simulink model "pid_ctrl_sim"  (R2015a)
settings: Solver=ode45  StartTime=0.0  StopTime=6  RelTol=1e-3
libraries: simulink x1
settings Model: Creator=rojas-j  LastModifiedBy=root

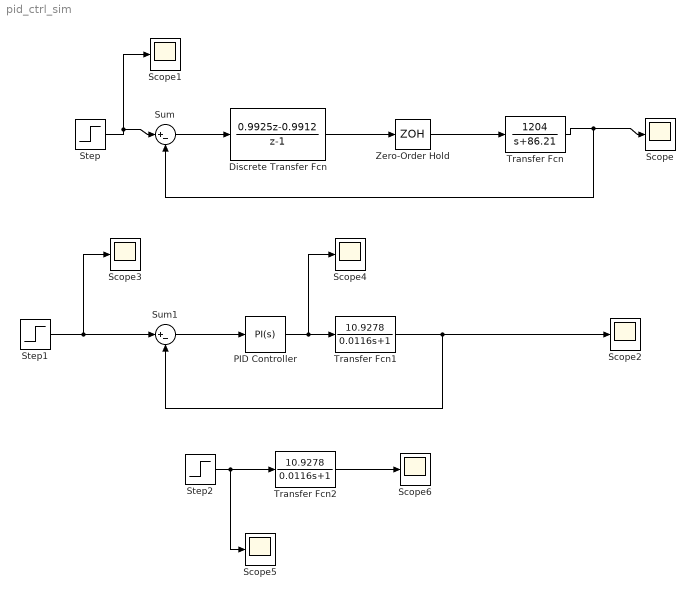
== system pid_ctrl_sim ==
  Discrete Transfer Fcn : DiscreteTransferFcn  Numerator=[0.9925,-0.9912]  Denominator=[1, -1]  SampleTime=0.00116
  PID Controller : simulink/Continuous/PID Controller  Controller=PI  TimeDomain=Continuous-time  SampleTime=-1  IntegratorMethod=Forward Euler  FilterMethod=Forward Euler  Form=Parallel  UseFilter=on  ControllerParametersSource=internal  P=0.99  I=1.17  D=0  N=100  InitialConditionSource=internal  InitialConditionForIntegrator=0  InitialConditionForFilter=0  ExternalReset=none  LimitOutput=off  UpperSaturationLimit=100  LowerSaturationLimit=0  LinearizeAsGain=on  AntiWindupMode=none  Kb=1  TrackingMode=off  Kt=1  PParamMin=[]  PParamMax=[]  IParamMin=[]  IParamMax=[]  DParamMin=[]  DParamMax=[]  NParamMin=[]  NParamMax=[]  KbParamMin=[]  KbParamMax=[]  KtParamMin=[]  KtParamMax=[]  POutMin=[]  POutMax=[]  IOutMin=[]  IOutMax=[]  DOutMin=[]  DOutMax=[]  NOutMin=[]  NOutMax=[]  KbOutMin=[]  KbOutMax=[]  KtOutMin=[]  KtOutMax=[]  IntegratorOutMin=[]  IntegratorOutMax=[]  FilterOutMin=[]  FilterOutMax=[]  SumOutMin=[]  SumOutMax=[]  SumI1OutMin=[]  SumI1OutMax=[]  SumI2OutMin=[]  SumI2OutMax=[]  SumI3OutMin=[]  SumI3OutMax=[]  SumDOutMin=[]  SumDOutMax=[]  SaturationOutMin=[]  SaturationOutMax=[]  IntegratorContinuousStateAttributes=''  IntegratorStateMustResolveToSignalObject=off  IntegratorRTWStateStorageClass=Auto  FilterContinuousStateAttributes=''  FilterStateMustResolveToSignalObject=off  FilterRTWStateStorageClass=Auto  DifferentiatorICPrevScaledInput=0  DifferentiatorOutMin=[]  DifferentiatorOutMax=[]
  Scope{,1..6} (7 alike) : Scope
      Scope2 settings: YMin=-1  YMax=1  SaveName=ScopeData2
      Scope3 settings: SaveName=ScopeData3
      Scope4 settings: YMin=-1  YMax=1  SaveName=ScopeData4
      Scope5 settings: SaveName=ScopeData5
      Scope6 settings: YMin=-1  YMax=1  SaveName=ScopeData6
  Step : Step  SampleTime=0.1
  Step1 : Step  After=500  SampleTime=0.1
  Step2 : Step  After=50  SampleTime=0.1
  Sum : Sum  Inputs=|+-
  Sum1 : Sum  Inputs=|+-
  Transfer Fcn : TransferFcn  Numerator=[1204]  Denominator=[1 86.21]
  Transfer Fcn1 : TransferFcn  Numerator=[10.9278]  Denominator=[0.0116 1]
  Transfer Fcn2 : TransferFcn  Numerator=[10.9278]  Denominator=[0.0116 1]
  Zero-Order Hold : ZeroOrderHold  SampleTime=0.00116
  wires:
  Step/1 -> Scope1/1, Sum/1
  Sum/1 -> Discrete Transfer Fcn/1
  Discrete Transfer Fcn/1 -> Zero-Order Hold/1
  Zero-Order Hold/1 -> Transfer Fcn/1
  Transfer Fcn/1 -> Sum/2, Scope/1
  Step1/1 -> Scope3/1, Sum1/1
  Sum1/1 -> PID Controller/1
  PID Controller/1 -> Scope4/1, Transfer Fcn1/1
  Transfer Fcn1/1 -> Scope2/1, Sum1/2
  Step2/1 -> Scope5/1, Transfer Fcn2/1
  Transfer Fcn2/1 -> Scope6/1
